simulink model "vehicle_animation"  (R2017b)
settings: Solver=FixedStepDiscrete  StartTime=0.0  StopTime=10000  FixedStep=.1  RelTol=1e-3  EnableMultiTasking=on
undefined symbols (not defined in the file or in its folder): drawVehicle
libraries: simulink x6
settings Model: Creator=beard  LastModifiedBy=mouse
settings DataIOCC: LimitDataPoints=on  SaveFormat=Array  SignalLoggingSaveFormat=ModelDataLogs
settings OptimizationCC: ExpressionDepthLimit=2147483647  InitFltsAndDblsToZero=on  LifeSpan=inf
settings DebuggingCC: UnderspecifiedInitializationDetection=Classic  MergeDetectMultiDrivingBlocksExec=none  SolverPrmCheckMsg=warning  FcnCallInpInsideContextMsg=warning  StateNameClashWarn=warning  SFUnexpectedBacktrackingDiag=warning  SFNoUnconditionalDefaultTransitionDiag=warning  SFExecutionAtInitializationDiag=none
settings HardwareCC: ProdBitPerPointer=32  ProdBitPerSizeT=32  ProdBitPerPtrDiffT=32  ProdLargestAtomicFloat=None  ProdIntDivRoundTo=Undefined  ProdEndianess=Unspecified  ProdWordSize=32  ProdHWDeviceType=32-bit Generic
settings ModelReferenceCC: PropagateSignalLabelsOutOfModel=off
settings CodeAppCC: StateflowObjectComments=on
settings GRTTargetCC: TargetLangStandard=C89/C90 (ANSI)  GeneratePreprocessorConditionals=Disable all  CombineOutputUpdateFcns=off  GRTInterface=on
settings ConfigComp: CovMetricSettings=dw  CovHtmlReporting=on  CovSaveCumulativeToWorkspaceVar=on  CovSaveSingleToWorkspaceVar=on  CovExternalEMLEnable=off  CovSFcnEnable=off

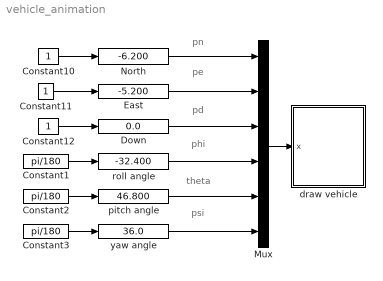
== system vehicle_animation ==
  note: pn
  note: pe
  note: pd
  note: phi
  note: theta
  note: psi
  Constant1 : Constant  Value=pi/180
  Constant10 : Constant
  Constant11 : Constant
  Constant12 : Constant
  Constant2 : Constant  Value=pi/180
  Constant3 : Constant  Value=pi/180
  Down : simulink/Math Operations/Slider Gain  gain=0.0  low=-10  high=10
  East : simulink/Math Operations/Slider Gain  gain=-5.200  low=-10  high=10
  Mux : Mux  Inputs=6
  North : simulink/Math Operations/Slider Gain  gain=-6.200  low=-10  high=10
  draw vehicle : Subsystem
      mask Display: image(imread('tv.jpg'))
  pitch angle : simulink/Math Operations/Slider Gain  gain=46.800  low=-180  high=180
  roll angle : simulink/Math Operations/Slider Gain  gain=-32.400  low=-180  high=180
  "yaw angle " : simulink/Math Operations/Slider Gain  gain=36.0  low=-180  high=180
  wires:
  Mux/1 -> draw vehicle/1(x)
  roll angle/1 -> Mux/4
  Constant1/1 -> roll angle/1
  Constant2/1 -> pitch angle/1
  "yaw angle "/1 -> Mux/6
  Constant3/1 -> "yaw angle "/1
  North/1 -> Mux/1
  Constant10/1 -> North/1
  East/1 -> Mux/2
  Constant11/1 -> East/1
  Down/1 -> Mux/3
  Constant12/1 -> Down/1
  pitch angle/1 -> Mux/5

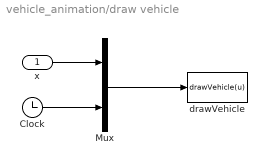
== system vehicle_animation/draw vehicle ==
  x : Inport
  Clock : Clock
  Mux : Mux  Inputs=2
  drawVehicle : MATLABFcn  MATLABFcn=drawVehicle(u)  OutputDimensions=0  SampleTime=0.1
  wires:
  Mux/1 -> drawVehicle/1
  x/1 -> Mux/1
  Clock/1 -> Mux/2
